simulink model "hnn_matrix_with_cost"  (R2024b)
settings: Solver=VariableStepAuto  StartTime=0.0  StopTime=10  RelTol=1e-3
settings Model: Creator=merlin  LastModifiedBy=merlin

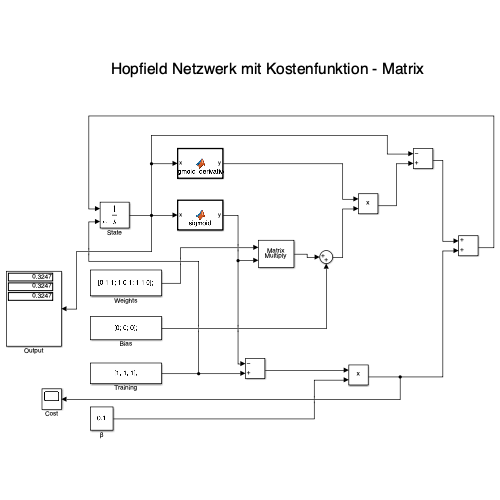
[thumbnail: Simulink's stored preview of the top-level diagram]
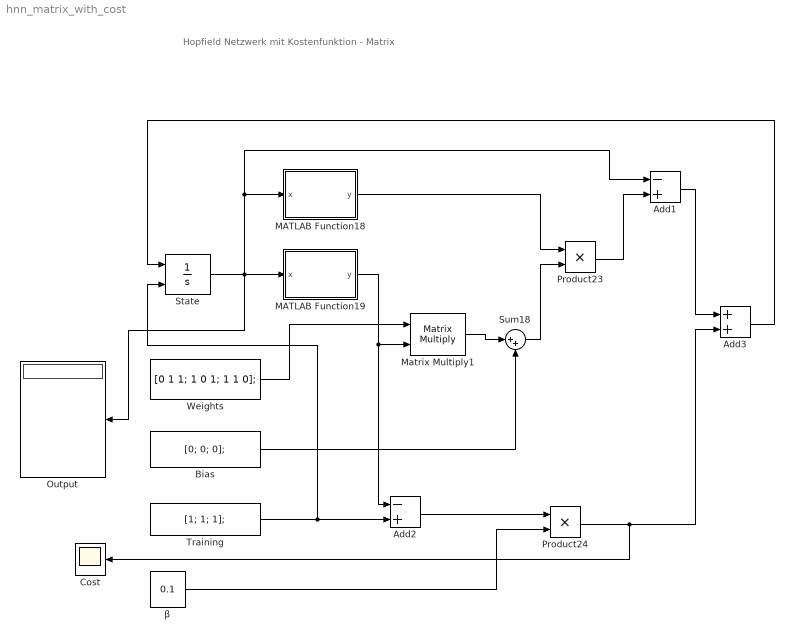
== system hnn_matrix_with_cost ==
  note: Hopfield Netzwerk mit Kostenfunktion - Matrix
  Add1 : Sum  Inputs=-+
  Add2 : Sum  Inputs=-+
  Add3 : Sum
  Bias : Constant  Value=[0; 0; 0];  VectorParams1D=off
  Cost : Scope
  MATLAB Function18 : MATLAB Function  TreatAsAtomicUnit=on
  MATLAB Function19 : MATLAB Function  TreatAsAtomicUnit=on
  Matrix Multiply1 : Product  Multiplication=Matrix(*)
  Output : Display
  Product23 : Product
  Product24 : Product
  State : Integrator  InitialConditionSource=external
  Sum18 : Sum  Inputs=|++
  Training : Constant  Value=[1; 1; 1];  VectorParams1D=off
  Weights : Constant  Value=[0 1 1; 1 0 1; 1 1 0];  VectorParams1D=off
  β : Constant  Value=0.1  VectorParams1D=off
  wires:
  Matrix Multiply1/1 -> Sum18/1
  State/1 -> MATLAB Function18/1(x), Add1/1, Output/1, MATLAB Function19/1(x)
  Weights/1 -> Matrix Multiply1/1
  Add1/1 -> Add3/1
  Bias/1 -> Sum18/2
  β/1 -> Product24/2
  Training/1 -> State/2, Add2/2
  Sum18/1 -> Product23/2
  Add3/1 -> State/1
  Product23/1 -> Add1/2
  Product24/1 -> Cost/1, Add3/2
  MATLAB Function19/1(y) -> Add2/1, Matrix Multiply1/2
  MATLAB Function18/1(y) -> Product23/1
  Add2/1 -> Product24/1

== matlab function hnn_matrix_with_cost/MATLAB Function19 ==
  data: x input; y output
function y = sigmoid(x)
y = 1 ./ (1 + exp(-x));
end

== matlab function hnn_matrix_with_cost/MATLAB Function18 ==
  data: x input; y output
function y = sigmoid_derivative(x)
sigmoid = 1 ./ (1 + exp(-x));
y = sigmoid .* (1 - sigmoid);
end
